simulink model "a2sw_nl_ged_demux"  (R2020b)
settings: Solver=ode45  StartTime=0.0  StopTime=30.0  MaxStep=0.01  RelTol=1e-3  EnableMultiTasking=on
model workspace (MAT data in the model file):
  c = 0.1
  delta = 0.1
  k = 1
  m = 2
  v0 = 0
  y0 = 2
settings Model: Creator=Reichl  LastModifiedBy=jakob
settings DataIOCC: LimitDataPoints=on  SaveFormat=Array  SignalLoggingSaveFormat=ModelDataLogs  ReturnWorkspaceOutputs=off
settings OptimizationCC: ExpressionDepthLimit=2147483647  LifeSpan=inf
settings DebuggingCC: UnderspecifiedInitializationDetection=Classic  MergeDetectMultiDrivingBlocksExec=none  SolverPrmCheckMsg=warning  FcnCallInpInsideContextMsg=warning  StateNameClashWarn=warning  SFUnexpectedBacktrackingDiag=warning  SFNoUnconditionalDefaultTransitionDiag=warning  SFExecutionAtInitializationDiag=none  ArithmeticOperatorsInVariantConditions=warning
settings HardwareCC: ProdBitPerPointer=32  ProdBitPerSizeT=32  ProdBitPerPtrDiffT=32  ProdLargestAtomicFloat=None  ProdIntDivRoundTo=Undefined  ProdEndianess=Unspecified  ProdWordSize=32  ProdHWDeviceType=32-bit Generic
settings ModelReferenceCC: PropagateSignalLabelsOutOfModel=off
settings SFSimCC: SimUseLocalCustomCode=off  CustomCodeUndefinedFunction=UseInterfaceOnly
settings RTWCC: RTWUseLocalCustomCode=off
settings CodeAppCC: StateflowObjectComments=on
settings GRTTargetCC: TargetLangStandard=C89/C90 (ANSI)  CombineOutputUpdateFcns=off  GRTInterface=on
settings ConfigComp: CovMetricSettings=dw  CovSaveCumulativeToWorkspaceVar=on  CovSaveSingleToWorkspaceVar=on  CovExternalEMLEnable=off  CovSFcnEnable=off

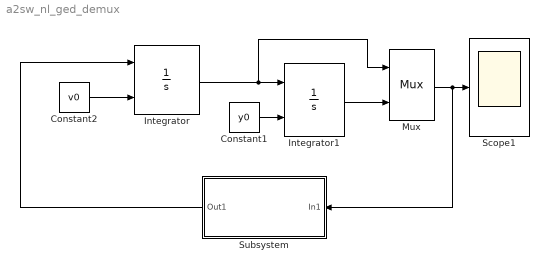
== system a2sw_nl_ged_demux ==
  " Constant2" : Constant  Value=v0
  Constant1 : Constant  Value=y0
  Integrator : Integrator  InitialConditionSource=external
  Integrator1 : Integrator  InitialConditionSource=external  InitialCondition=3
  Mux : Mux  Inputs=2
  Scope1 : Scope
  Subsystem : Subsystem
  wires:
  Integrator/1 -> Integrator1/1, Mux/1
  " Constant2"/1 -> Integrator/2
  Constant1/1 -> Integrator1/2
  Subsystem/1(Out1) -> Integrator/1
  Integrator1/1 -> Mux/2
  Mux/1 -> Scope1/1, Subsystem/1(In1)

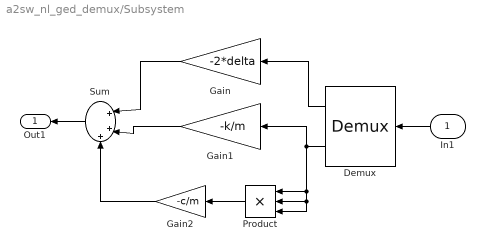
== system a2sw_nl_ged_demux/Subsystem ==
  In1 : Inport
  Demux : Demux  Outputs=2
      settings: DisplayOption=none
  Gain : Gain  Gain=-2*delta
  Gain1 : Gain  Gain=-k/m
  Gain2 : Gain  Gain=-c/m
  Product : Product  Inputs=3
  Sum : Sum  Inputs=|+++
  Out1 : Outport  VectorParamsAs1DForOutWhenUnconnected=off
  wires:
  Sum/1 -> Out1/1
  Gain/1 -> Sum/1
  Gain1/1 -> Sum/2
  Demux/1 -> Gain/1
  Demux/2 -> Gain1/1, Product/1, Product/3, Product/2
  In1/1 -> Demux/1
  Product/1 -> Gain2/1
  Gain2/1 -> Sum/3
